simulink model "MACARAIG_SIMULINK_NO5"  (R2024a)
settings: Solver=VariableStepAuto  StartTime=0.0  StopTime=20  RelTol=1e-3
values from neighbouring files (symbols this model uses):
  g5_den = [b7, b6,b5,b4, b3, b2, b1, b]    [LAB 2 NO. 5 AND NO. 6.m]
  G5_num = [a7, a6, a5,a4,a3,a2,a]    [LAB 2 NO. 5 AND NO. 6.m]

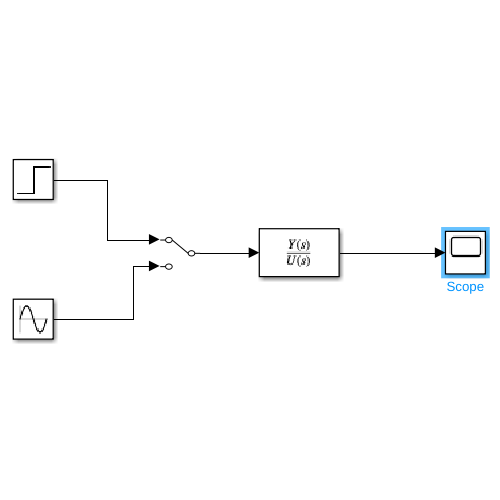
[thumbnail: Simulink's stored preview of the top-level diagram]
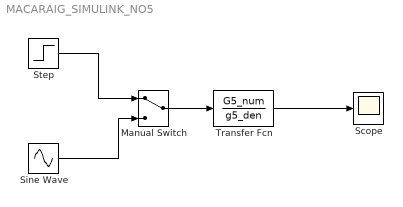
== system MACARAIG_SIMULINK_NO5 ==
  Manual Switch : ManualSwitch
  Scope : Scope
  Sine Wave : Sin  SampleTime=0
  Step : Step  Time=0  SampleTime=0
  Transfer Fcn : TransferFcn  Numerator=G5_num  Denominator=g5_den
  wires:
  Step/1 -> Manual Switch/1
  Sine Wave/1 -> Manual Switch/2
  Manual Switch/1 -> Transfer Fcn/1
  Transfer Fcn/1 -> Scope/1
